simulink model "DCC_DTC_v5"  (R2023b)
settings: Solver=FixedStepDiscrete  StartTime=0.0  StopTime=0.4  MaxStep=1e-  RelTol=1e-6
undefined symbols (not defined in the file): DiscIntNeverNeededParam
libraries: spsPermanentMagnetSynchronousMachineLib x3, simulink x2, spsDCVoltageSourceLib x1, spsGroundLib x1, slpidlib x1, spsThreePhaseVIMeasurementLib x1, spsUniversalBridgeLib x1, sps_lib x1
settings Model: Creator=rainy  LastModifiedBy=rainy
settings DataIOCC: ReturnWorkspaceOutputs=off

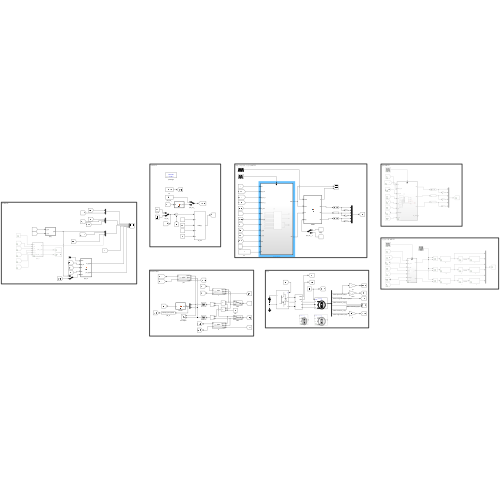
[thumbnail: Simulink's stored preview of the top-level diagram]
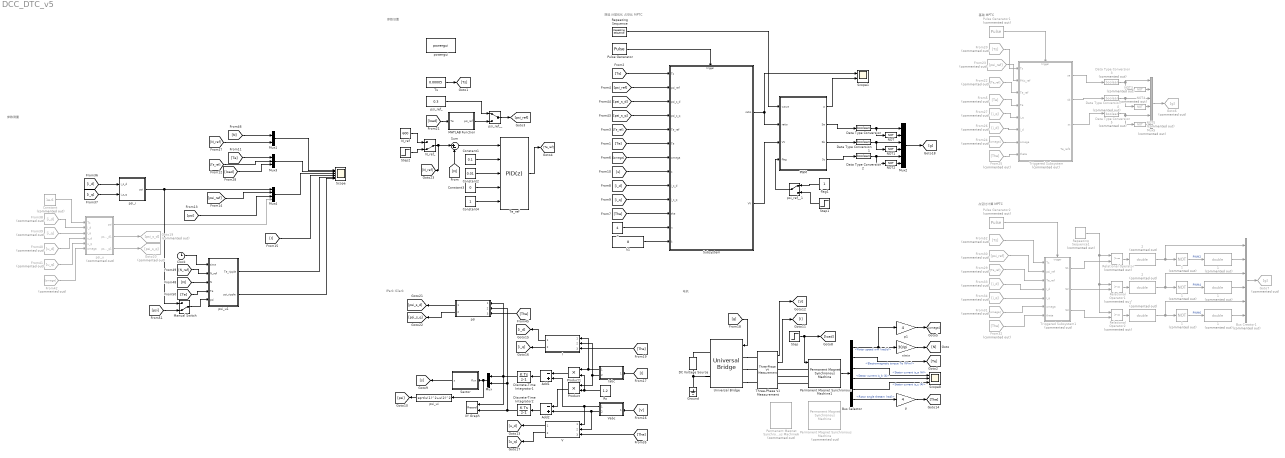
== system DCC_DTC_v5 ==
  note: 参数设置
  note: 参数测量
  note: IPark IClark
  note: 电机
  note: 基础 MPTC
  note: 占空比计算 MPTC
  note: 筛选 分层优化 占空比 MPTC
  "         1" : DataTypeConversion  Commented=on  OutDataTypeStr=double  SaturateOnIntegerOverflow=off  RndMeth=Floor
  "         2" : DataTypeConversion  Commented=on  OutDataTypeStr=double  SaturateOnIntegerOverflow=off  RndMeth=Floor
  "       1" : Logic  Commented=on  Operator=NOT  AllPortsSameDT=off  OutDataTypeStr=boolean
  "     1" : DataTypeConversion  Commented=on  OutDataTypeStr=double  SaturateOnIntegerOverflow=off  RndMeth=Floor
  "     2" : DataTypeConversion  Commented=on  OutDataTypeStr=double  SaturateOnIntegerOverflow=off  RndMeth=Floor
  "   1" : Logic  Commented=on  Operator=NOT  AllPortsSameDT=off  OutDataTypeStr=boolean
  "  1" : DataTypeConversion  Commented=on  OutDataTypeStr=double  SaturateOnIntegerOverflow=off  RndMeth=Floor
  "  2" : DataTypeConversion  Commented=on  OutDataTypeStr=double  SaturateOnIntegerOverflow=off  RndMeth=Floor
  " 1" : Logic  Commented=on  Operator=NOT  AllPortsSameDT=off  OutDataTypeStr=boolean
  Add1 : Sum  Inputs=-+
  Add2 : Sum  Inputs=-+
  Bus Creator1 : BusCreator  Commented=on  Inputs=6
  Bus Selector : BusSelector  OutputSignals=Rotor speed wm (rad/s),Electromagnetic torque Te (N*m),Stator current is_a (A),Stator current is_b (A),Stator current is_c (A),Rotor angle thetam (rad)
  Clock : Clock
  Constant : Constant  Commented=on  Value=1e-6
  Constant1 : Constant  Value=0.1
  Constant2 : Constant  Value=0.01
  Constant3 : Constant  Value=0
  Constant4 : Constant
  DC Voltage Source : spsDCVoltageSourceLib/DC Voltage Source  Amplitude=311  Measurements=Voltage
  Data Type Conversion : DataTypeConversion  OutDataTypeStr=boolean  SaturateOnIntegerOverflow=off  RndMeth=Floor
  Data Type Conversion1 : DataTypeConversion  OutDataTypeStr=boolean  SaturateOnIntegerOverflow=off  RndMeth=Floor
  Data Type Conversion2 : DataTypeConversion  OutDataTypeStr=boolean  SaturateOnIntegerOverflow=off  RndMeth=Floor
  Data Type Conversion3 : DataTypeConversion  Commented=on  OutDataTypeStr=boolean  SaturateOnIntegerOverflow=off  RndMeth=Floor
  Data Type Conversion4 : DataTypeConversion  Commented=on  OutDataTypeStr=boolean  SaturateOnIntegerOverflow=off  RndMeth=Floor
  Data Type Conversion5 : DataTypeConversion  Commented=on  OutDataTypeStr=boolean  SaturateOnIntegerOverflow=off  RndMeth=Floor
  Discrete-Time Integrator1 : DiscreteIntegrator  SampleTime=-1  ICPrevOutput=DiscIntNeverNeededParam  ICPrevScaledInput=DiscIntNeverNeededParam
  Discrete-Time Integrator2 : DiscreteIntegrator  SampleTime=-1  ICPrevOutput=DiscIntNeverNeededParam  ICPrevScaledInput=DiscIntNeverNeededParam
  From20 : From  Commented=on  GotoTag=Ts
  From22 : From  Commented=on  GotoTag=Te_ref
  From23 : From  Commented=on  GotoTag=psi_ref
  From24 : From  Commented=on  GotoTag=omega
  From25 : From  Commented=on  GotoTag=The
  From26 : From  Commented=on  GotoTag=i_d
  From27 : From  Commented=on  GotoTag=i_q
  From29 : From  Commented=on  GotoTag=Te_ref
  From30 : From  Commented=on  GotoTag=psi_ref
  From31 : From  Commented=on  GotoTag=omega
  From32 : From  Commented=on  GotoTag=The
  From33 : From  Commented=on  GotoTag=i_d
  From34 : From  Commented=on  GotoTag=i_q
  From38 : From  Commented=on  GotoTag=i_d
  From39 : From  Commented=on  GotoTag=i_q
  From40 : From  Commented=on  GotoTag=u_d
  From41 : From  Commented=on  GotoTag=u_q
  From42 : From  Commented=on  GotoTag=omega
  From5 : From  Commented=on  GotoTag=Te
  From52 : From  Commented=on  GotoTag=Ts
  Goto19 : Goto  Commented=on  GotoTag=psi_s_d
  Goto20 : Goto  Commented=on  GotoTag=psi_s_q
  Goto6 : Goto  Commented=on  GotoTag=g
  Goto7 : Goto  Commented=on  GotoTag=g
  Ground : spsGroundLib/Ground  LConnTagsString=a
  I : Subsystem  ReferencedSubsystem=Park
  Iabc : Subsystem  ReferencedSubsystem=Clark
  MATLAB Function : MATLAB Function  TreatAsAtomicUnit=on
  Manual Switch : ManualSwitch  CurrentSetting=0
  Mux : Mux  Inputs=2
  Mux1 : Mux  Inputs=2
  Mux2 : Mux  Inputs=6
  Mux3 : Mux  Inputs=3
  Mux4 : Mux
  Mux5 : Mux  Commented=on  Inputs=6
  NOT : Logic  Operator=NOT  IconShape=distinctive  AllPortsSameDT=off  OutDataTypeStr=boolean
  NOT1 : Logic  Operator=NOT  IconShape=distinctive  AllPortsSameDT=off  OutDataTypeStr=boolean
  NOT2 : Logic  Operator=NOT  IconShape=distinctive  AllPortsSameDT=off  OutDataTypeStr=boolean
  NOT3 : Logic  Commented=on  Operator=NOT  IconShape=distinctive  AllPortsSameDT=off  OutDataTypeStr=boolean
  NOT4 : Logic  Commented=on  Operator=NOT  IconShape=distinctive  AllPortsSameDT=off  OutDataTypeStr=boolean
  NOT5 : Logic  Commented=on  Operator=NOT  IconShape=distinctive  AllPortsSameDT=off  OutDataTypeStr=boolean
  N_ref : Constant  Value=600
  N_ref_ : ManualSwitch  CurrentSetting=0
  PWM : MATLAB Function  TreatAsAtomicUnit=on
  Permanent Magnet Synchronous Machine : spsPermanentMagnetSynchronousMachineLib/Permanent Magnet Synchronous Machine  Commented=on  NbPhases=3  FluxDistribution=Sinusoidal  RotorType=Salient-pole  MechanicalLoad=Torque Tm  PresetModel="02:  1.7 Nm 300 Vdc 3750 RPM - 1.7 Nm"  ShowDetailedParameters=on  MeasurementBus=off  Resistance=4.765  Inductance=8.5e-3  dqInductances=[0.0133 0.0147]  La=0.0005  MachineConstant=Flux linkage established by magnets (V.s)  Flux=0.1848  VoltageCst=67.038  TorqueCst=0.5544  Flat=120  Mechanical=[0.0001051 4.047e-05 2 0]  PolePairs=2  InitialConditions=[0 0 0 0]  InitialConditions5ph=[0 0 0 0 0 0]  RefAngle=Aligned with phase A axis (original Park)  IterativeDiscreteModel=Trapezoidal non iterative  TsBlock=-1  TsPowergui=0
  Permanent Magnet Synchronous Machine1 : spsPermanentMagnetSynchronousMachineLib/Permanent Magnet Synchronous Machine  NbPhases=3  FluxDistribution=Sinusoidal  RotorType=Round  MechanicalLoad=Torque Tm  PresetModel=No  ShowDetailedParameters=on  MeasurementBus=off  Resistance=1.2  Inductance=8.5e-3  dqInductances=[8.5e-3,8.5e-3]  La=8.5e-3  MachineConstant=Flux linkage established by magnets (V.s)  Flux=0.175  VoltageCst=126.966  TorqueCst=1.05  Flat=120  Mechanical=[0.0008 0.0004924 4 0]  PolePairs=4  InitialConditions=[0,0, 0,0]  InitialConditions5ph=[0 0 0 0 0 0]  RefAngle=Aligned with phase A axis (original Park)  IterativeDiscreteModel=Trapezoidal non iterative  TsBlock=-1  TsPowergui=0
  Permanent Magnet Synchronous Machine6 : spsPermanentMagnetSynchronousMachineLib/Permanent Magnet Synchronous Machine  Commented=on  NbPhases=3  FluxDistribution=Sinusoidal  RotorType=Round  MechanicalLoad=Torque Tm  PresetModel=No  ShowDetailedParameters=on  MeasurementBus=off  Resistance=0.25  Inductance=8.5e-3  dqInductances=[8.5e-3,8.5e-3]  La=0.0005  MachineConstant=Flux linkage established by magnets (V.s)  Flux=0.01325  VoltageCst=9.6131  TorqueCst=0.0795  Flat=120  Mechanical=[0.00003 0 4 0]  PolePairs=4  InitialConditions=[0,0, 0,0]  InitialConditions5ph=[0 0 0 0 0 0]  RefAngle=Aligned with phase A axis (original Park)  IterativeDiscreteModel=Trapezoidal non iterative  TsBlock=-1  TsPowergui=0
  Product : Product
  Product1 : Product
  Pulse Generator : DiscretePulseGenerator  PulseType=Time based  Period=0.00005
  Pulse Generator1 : DiscretePulseGenerator  Commented=on  PulseType=Time based  Period=0.00005
  Pulse Generator2 : DiscretePulseGenerator  Commented=on  PulseType=Time based  Period=0.00005
  Relational Operator : RelationalOperator  Commented=on  OutDataTypeStr=boolean  RndMeth=Simplest  InputSameDT=off
  Relational Operator1 : RelationalOperator  Commented=on  OutDataTypeStr=boolean  RndMeth=Simplest  InputSameDT=off
  Relational Operator2 : RelationalOperator  Commented=on  OutDataTypeStr=boolean  RndMeth=Simplest  InputSameDT=off
  Repeating Sequence : simulink/Sources/Repeating Sequence  rep_seq_t=[0 0.000025 0.00005]  rep_seq_y=[0 1 0]
  Repeating Sequence1 : simulink/Sources/Repeating Sequence  Commented=on  rep_seq_t=[0 0.000025 0.00005]  rep_seq_y=[0 0.000025 0]
  Rs : Constant  Value=1.2
  Scope : Scope  NumInputPorts=6
  Scope1 : Scope  NumInputPorts=2
  Scope8 : Scope  NumInputPorts=3
  Sector : MATLAB Function  TreatAsAtomicUnit=on
  Step : Step  Time=0.2  After=0  SampleTime=0
  Step1 : Step  Time=0.1  SampleTime=0
  Step2 : Step  Time=0.2  Before=400  After=600  SampleTime=0
  Subsystem : Subsystem
  Sum : Sum  Inputs=|+-
  Te_ref : slpidlib/PID Controller  Controller=PID  Form=Parallel  TimeDomain=Discrete-time  UseExternalTs=off  SampleTime=-1  IntegratorMethod=Forward Euler  FilterMethod=Forward Euler  ControllerParametersSource=external  P=1  I=1  UseKiTs=off  D=0  N=100  UseFilter=on  TunerSelectOption=Transfer Function Based (PID Tuner App)  InitialConditionSource=internal  InitialConditionForIntegrator=0  InitialConditionForFilter=0  DifferentiatorICPrevScaledInput=0  ExternalReset=none  TrackingMode=off  Kt=1  LimitOutput=off  SatLimitsSource=internal  UpperSaturationLimit=inf  LowerSaturationLimit=-inf  LinearizeAsGain=off  AntiWindupMode=none  Kb=1  LimitIntegrator=off  UpperIntegratorSaturationLimit=inf  LowerIntegratorSaturationLimit=-inf  POutMin=[]  POutMax=[]  IOutMin=[]  IOutMax=[]  DOutMin=[]  DOutMax=[]  NOutMin=[]  NOutMax=[]  SumOutMin=[]  SumOutMax=[]  SaturationOutMin=[]  SaturationOutMax=[]  PParamMin=[]  PParamMax=[]  IParamMin=[]  IParamMax=[]  DParamMin=[]  DParamMax=[]  NParamMin=[]  NParamMax=[]  KbParamMin=[]  KbParamMax=[]  KtParamMin=[]  KtParamMax=[]  KbOutMin=[]  KbOutMax=[]  KtOutMin=[]  KtOutMax=[]  IntegratorOutMin=[]  IntegratorOutMax=[]  FilterOutMin=[]  FilterOutMax=[]  SumI1OutMin=[]  SumI1OutMax=[]  SumI2OutMin=[]  SumI2OutMax=[]  SumI3OutMin=[]  SumI3OutMax=[]  SumI4OutMin=[]  SumI4OutMax=[]  SumDOutMin=[]  SumDOutMax=[]  DifferentiatorOutMin=[]  DifferentiatorOutMax=[]  FilterDiffOutCoefMin=[]  FilterDiffOutCoefMax=[]  ReciprocalOutMin=[]  ReciprocalOutMax=[]  SumDenOutMin=[]  SumDenOutMax=[]  SumNumOutMin=[]  SumNumOutMax=[]  DivideOutMin=[]  DivideOutMax=[]  UdiffTsProdOutMin=[]  UdiffTsProdOutMax=[]  NTsProdOutMin=[]  NTsProdOutMax=[]  UintegralTsProdOutMin=[]  UintegralTsProdOutMax=[]  UngainTsProdOutMin=[]  UngainTsProdOutMax=[]  ClampingZeroOutDataTypeStr=Inherit: Inherit via back propagation  ClampingZeroOutMin=[]  ClampingZeroOutMax=[]  FilterDenConstantOutDataTypeStr=Inherit: Inherit via back propagation  FilterDenConstantOutMin=[]  FilterDenConstantOutMax=[]  PCopyOutDataTypeStr=Inherit: Inherit via back propagation  PCopyOutMin=[]  PCopyOutMax=[]  NCopyOutDataTypeStr=Inherit: Inherit via back propagation  NCopyOutMin=[]  NCopyOutMax=[]  IntegratorContinuousStateAttributes=''  IntegratorStateMustResolveToSignalObject=off  IntegratorRTWStateStorageClass=Auto  FilterContinuousStateAttributes=''  FilterStateMustResolveToSignalObject=off  FilterRTWStateStorageClass=Auto  ParallelPVariant=ExternalParameters  IdealPVariant=Disabled  IVariant=ExternalParameters  DVariant=ExternalParameters  IntegratorVariant=Discrete  SatVariant=Disabled  AWVariant=Passthrough  PCopyVariant=Disabled  TRVariant=Disabled  FdbkBlocksVariant=Forward  IdealPFdbkVariant=Disabled  SatFdbkVariant=Disabled  DerivativeFilterVariant=ForwardEulerFilter  NVariant=ExternalParameters  NCopyVariant=Disabled  FilterICVariant=InternalICsFilter  IntegratorICVariant=InternalICs  ExternalResetVariant=Disabled  TRSumVariant=Passthrough  SumFdbkVariant=Disabled  SumVariant=Sum_PID  TsampFilterVariant=InternalTs  TsampNgainVariant=Passthrough  TsampIntegralVariant=Disabled_SignalSpec  ExternalSaturationOutDataTypeStr=Inherit: Same as second input
      settings: LibrarySourceBlock=simulink/Discrete/Discrete PID Controller
  Three-Phase V-I Measurement : spsThreePhaseVIMeasurementLib/Three-Phase V-I Measurement  VoltageMeasurement=phase-to-ground  SetLabelV=off  LabelV=Vabc  Vpu=off  VpuLL=off  CurrentMeasurement=yes  SetLabelI=off  LabelI=Iabc  Ipu=off  Pbase=100e6  Vbase=500e3  OutputType=Complex  PhasorSimulation=off  PSBequivalent=0
  Triggered Subsystem : Subsystem  Commented=on  TreatAsAtomicUnit=on
  Triggered Subsystem1 : Subsystem  Commented=on  TreatAsAtomicUnit=on
  Ts : Constant  Value=0.00005
  Universal Bridge : spsUniversalBridgeLib/Universal Bridge  Arms=3  SnubberResistance=1e5  SnubberCapacitance=inf  Device=IGBT / Diodes  Ron=1e-3  Lon=0  ForwardVoltages="[  0  0  ]"  ForwardVoltage=0  GTOparameters=[ 10e-6 , 20e-6 ]  IGBTparameters=[ 1e-6 , 2e-6 ]  Measurements=None  Measurements_2=None  converterType=Rectifier
  V : Subsystem  ReferencedSubsystem=Park
  Vabc : Subsystem  ReferencedSubsystem=Clark
  XY Graph : Record  FileSettingsInternal="{\"entries\":[{\"content\":{\"excelSettings\":{\"content\":{},\"type\":\"Streamout.ExcelSettings\"}},\"type\":\"Streamout.FileSettingStorage\",\"uuid\":\"\"}],\"packageUris\":[\"http:\\/\\/schema.mathworks.com\\/mf0\\/streamout_blocks\\/R2020a\"],\"version\":\"1.0\"}"  Layout=[1 1]  SignalsInternal="{\"entries\":[{\"content\":{\"signals\":[{\"content\":{\"blockPath\":[],\"dimensions\":[1],\"domain\":\"\",\"lineColor\":\"#a2142f\",\"plots\":[1],\"port\":1,\"sid\":[\"\"],\"signalID\":316,\"signalName\":\"Discrete-Time\\nIntegrator1\"},\"type\":\"RecordBlkView.Signal\",\"uuid\":\"\"},{\"content\":{\"blockPath\":[],\"dimensions\":[1],\"domain\":\"\",\"lineColor\":\"#139fff\",\"plots\":[1],\"port\":2,\"sid\":[\"\"],\"signalID\":320,\"signalName\":\"Discrete-Time\\nIntegrator2\"},\"type\":\"RecordBlkView.Signal\",\"uuid\":\"\"}]},\"type\":\"RecordBlkView.InputSignals\",\"uuid\":\"\"}],\"packageUris\":[\"http:\\/\\/schema.mathworks.com\\/mf0\\/streamout_blocks\\/R2020a\"],\"version\":\"1.0\"}"  VisualizationBindings="{\"xyplotplugin\":{\"info\":[{\"series\":[{\"bindingParametersList\":[{\"parameter\":\"X-Axis\",\"signalID\":316,\"signalName\":\"Discrete-Time\\nIntegrator1\"},{\"parameter\":\"Y-Axis\",\"signalID\":320,\"signalName\":\"Discrete-Time\\nIntegrator2\"}],\"seriesID\":39498}],\"subplotID\":1}]}}"  CompatibilityTag=XY  st=-1
  flag1 : Constant
  k1 : Constant  Value=8
  n : Constant  Value=4
  p : Gain  Gain=4
  p1 : Gain  Gain=4
  powergui : sps_lib/powergui  Priority=1  SimulationMode=Discrete  SampleTime=1e-6  frequency=60  Iterations=50  frequencyindice=0  Pbase=100e6  ErrMax=1e-4  UnitsV=kV  UnitsW=MW  buscounter=0  FunctionMessages=off  echomessages=off  EnableUseOfTLC=off  CurrentSourceSwitches=off  DisableSnubberDevices=off  DisableRonSwitches=off  DisableVfSwitches=off  DisplayEquations=off  AutomaticDiscreteSolvers=off  SolverType=Tustin/Backward Euler (TBE)  Interpol=off  ExternalGateDelay=off  methode=off  Ts=100  x0status=blocks  SPID=on  SwTol=0  HookPort=off  NonlinearTolerance=1e-4  nMaxIteration=100  ContinueOnMaxIteration=off  RestoreLinks=warning  ResistiveCurrentMeasurement=off  Frange=[0:2:500]  Ylog=off  Xlog=on  ShowGrid=off  save=off  variable=ZData  structure=0  ZoomFFT=off  StartTime=0.0  cycles=1  DisplayStyle=1  fundamental=60  FreqAxis=off  MaxFrequency=1000  frequencyindicesteady=1  RmsSteady=1  display=off
  psi : Subsystem  ReferencedSubsystem=Park
  psi_i : MATLAB Function  TreatAsAtomicUnit=on
  psi_ref_ : Constant  Value=0.3
  psi_ref__ : ManualSwitch
  psi_ref__1 : ManualSwitch
  psi_u : MATLAB Function  Commented=on  TreatAsAtomicUnit=on
  psi_u1 : MATLAB Function  TreatAsAtomicUnit=on
  psi_ui : Fcn  Expr=sqrt(u(1)^2+u(2)^2)
  r/min : Gain  Gain=30/pi
  wires:
  N_ref_/1 -> [N_ref], Sum/1
  Sum/1 -> Te_ref/1
  Bus Selector/1 -> p1/1, r/min/1  "<Rotor speed wm (rad/s)>"
  r/min/1 -> [N]
  [N] -> Sum/2
  NOT1/1 -> Mux2/4
  Data Type Conversion2/1 -> NOT2/1, Mux2/5
  NOT2/1 -> Mux2/6
  Data Type Conversion/1 -> NOT/1, Mux2/1
  NOT/1 -> Mux2/2
  Data Type Conversion1/1 -> NOT1/1, Mux2/3
  Iabc/1 -> I/1, Product1/1
  Iabc/2 -> Product/1, I/2
  Rs/1 -> Product/2, Product1/2
  Product1/1 -> Add1/1
  Vabc/1 -> V/1, Add1/2
  Product/1 -> Add2/1
  Vabc/2 -> V/2, Add2/2
  Add2/1 -> Discrete-Time Integrator2/1
  Add1/1 -> Discrete-Time Integrator1/1
  Ts/1 -> [Ts]
  Mux/1 -> psi_ui/1, Sector/1(flux)
  Bus Selector/2 -> [Te]  "<Electromagnetic torque Te (N*m)>"
  [Te] -> Subsystem/6(Te)
  Three-Phase V-I Measurement/2 -> [I]
  PWM/4(Sc) -> Data Type Conversion2/1
  PWM/3(Sb) -> Data Type Conversion1/1
  PWM/2(Sa) -> Data Type Conversion/1
  [Ts] -> Subsystem/1(Ts)
  [psi_ref] -> Subsystem/2(psi_ref)
  Repeating Sequence/1 -> PWM/1(wave)
  Pulse Generator/1 -> Subsystem/Trigger
  n/1 -> Subsystem/12(n)
  Bus Selector/3 -> Scope8/1  "<Stator current is_a (A)>"
  Bus Selector/4 -> Scope8/2  "<Stator current is_b (A)>"
  Bus Selector/5 -> Scope8/3  "<Stator current is_c (A)>"
  Step/1 -> Permanent Magnet Synchronous Machine1/1, [load]
  Subsystem/1(ratio) -> Scope1/1, PWM/2(ratio)
  Subsystem/2(VV) -> PWM/3(VV)
  Te_ref/1 -> [Te_ref]
  [Te_ref] -> Subsystem/5(Te_ref)
  [omega] -> Subsystem/7(omega)
  [i_d] -> Subsystem/9(i_s_d)
  [i_q] -> Subsystem/10(i_s_q)
  Sector/1(s) -> [s]
  [s] -> Subsystem/8(s)
  PWM/1(w) -> Scope1/2
  psi_ui/1 -> [psi]
  Mux1/1 -> Scope/1
  Mux3/1 -> Scope/2
  Mux4/1 -> Scope/3
  [I] -> Scope/4
  [Te] -> Mux3/1
  [psi_ref] -> Mux4/2
  Three-Phase V-I Measurement/1 -> [V]
  [I] -> Iabc/1
  [V] -> Vabc/1
  Mux2/1 -> [g]
  [g] -> Universal Bridge/1
  Bus Selector/6 -> p/1  "<Rotor angle thetam (rad)>"
  p/1 -> [The]
  [The] -> I/3
  I/2 -> [i_q]
  I/1 -> [i_d]
  p1/1 -> [omega]
  k1/1 -> Subsystem/13(k)
  Discrete-Time Integrator1/1 -> psi/1, XY Graph/1, Mux/1
  Discrete-Time Integrator2/1 -> XY Graph/2, psi/2, Mux/2
  [load] -> MATLAB Function/1(Te)
  psi_ref_/1 -> psi_ref__/1
  MATLAB Function/1(psi_ref) -> psi_ref__/2
  psi_ref__/1 -> [psi_ref]
  [i_d] -> psi_i/1(i_s_d)
  [i_q] -> psi_i/2(i_s_q)
  Permanent Magnet Synchronous Machine1/1 -> Bus Selector/1
  [psi] -> Mux4/3
  [The] -> Subsystem/11(the)
  NOT3/1 -> Mux5/2
  NOT4/1 -> Mux5/4
  NOT5/1 -> Mux5/6
  Triggered Subsystem/1(sa) -> Data Type Conversion3/1
  Data Type Conversion5/1 -> NOT5/1, Mux5/5
  Triggered Subsystem/2(sb) -> Data Type Conversion4/1
  Triggered Subsystem/3(sc) -> Data Type Conversion5/1
  Data Type Conversion3/1 -> NOT3/1, Mux5/1
  Data Type Conversion4/1 -> NOT4/1, Mux5/3
  Mux5/1 -> Goto6/1
  From25/1 -> Triggered Subsystem/8(theta)
  From24/1 -> Triggered Subsystem/7(omega)
  From26/1 -> Triggered Subsystem/6(i_d)
  From27/1 -> Triggered Subsystem/5(i_q)
  From5/1 -> Triggered Subsystem/4(Te)
  From22/1 -> Triggered Subsystem/3(Te_ref)
  From23/1 -> Triggered Subsystem/2(Phis_ref)
  From20/1 -> Triggered Subsystem/1(Ts)
  Pulse Generator1/1 -> Triggered Subsystem/Trigger
  [load] -> Mux3/3
  [Te_ref] -> Mux3/2
  flag1/1 -> psi_ref__1/1
  Step1/1 -> psi_ref__1/2
  psi_ref__1/1 -> PWM/4(flag)
  From30/1 -> Triggered Subsystem1/2(psi_ref)
  From29/1 -> Triggered Subsystem1/3(Te_ref)
  From34/1 -> Triggered Subsystem1/5(i_q)
  From33/1 -> Triggered Subsystem1/4(i_d)
  From31/1 -> Triggered Subsystem1/6(omega)
  From32/1 -> Triggered Subsystem1/7("theta ")
  [The] -> V/3
  V/1 -> [u_d]
  V/2 -> [u_q]
  Constant/1 -> psi_u/1(Ts)
  From40/1 -> psi_u/4(u_d)
  From41/1 -> psi_u/5(u_q)
  psi_u/1(psi) -> Mux4/4
  From42/1 -> psi_u/6(omega)
  psi_u/2(psi_s_d1) -> Goto19/1
  psi_u/3(psi_s_q1) -> Goto20/1
  [psi_s_d] -> Subsystem/3(psi_s_d)
  [psi_s_q] -> Subsystem/4(psi_s_q)
  psi/1 -> [psi_s_d]
  psi/2 -> [psi_s_q]
  [The] -> psi/3
  Constant1/1 -> Te_ref/2
  Constant2/1 -> Te_ref/3
  Constant3/1 -> Te_ref/4
  Constant4/1 -> Te_ref/5
  N_ref/1 -> N_ref_/1
  Step2/1 -> N_ref_/2
  [N_ref] -> Mux1/2
  [N] -> Mux1/1
  From39/1 -> psi_u/3(i_q)
  From38/1 -> psi_u/2(i_d)
  [N_ref] -> psi_u1/2(N_ref)
  [N] -> psi_u1/3(N)
  [Te] -> psi_u1/4(Te)
  psi_u1/1(Te_ripple) -> Scope/5
  psi_u1/2(psi_ripple) -> Scope/6
  From52/1 -> Triggered Subsystem1/1(Ts)
  Pulse Generator2/1 -> Triggered Subsystem1/Trigger
  Triggered Subsystem1/1(S1) -> Relational Operator/2
  Triggered Subsystem1/2(S2) -> Relational Operator1/2
  "  2"/1 -> Bus Creator1/1, " 1"/1
  Bus Creator1/1 -> Goto7/1
  Relational Operator/1 -> "  2"/1
  "         1"/1 -> Bus Creator1/6
  Relational Operator2/1 -> "         2"/1
  "       1"/1 -> "         1"/1  "PWM6"
  Relational Operator1/1 -> "     2"/1
  "   1"/1 -> "     1"/1  "PWM4"
  " 1"/1 -> "  1"/1  "PWM2"
  "  1"/1 -> Bus Creator1/2
  Repeating Sequence1/1 -> Relational Operator2/1, Relational Operator1/1, Relational Operator/1
  "         2"/1 -> Bus Creator1/5, "       1"/1
  "     1"/1 -> Bus Creator1/4
  "     2"/1 -> Bus Creator1/3, "   1"/1
  Triggered Subsystem1/3(S3) -> Relational Operator2/2
  Clock/1 -> psi_u1/1(time)
  Manual Switch/1 -> psi_u1/5(psi)
  [psi] -> Manual Switch/2
  psi_i/1(psi) -> Manual Switch/1, Mux4/1
  connections:
  Universal Bridge/RConn2 -- DC Voltage Source/LConn1 -- Ground/LConn1
  Universal Bridge/LConn3 -- Three-Phase V-I Measurement/LConn3
  Universal Bridge/LConn1 -- Three-Phase V-I Measurement/LConn1
  Universal Bridge/LConn2 -- Three-Phase V-I Measurement/LConn2
  DC Voltage Source/RConn1 -- Universal Bridge/RConn1
  Permanent Magnet Synchronous Machine1/LConn1 -- Three-Phase V-I Measurement/RConn1
  Permanent Magnet Synchronous Machine1/LConn2 -- Three-Phase V-I Measurement/RConn2
  Permanent Magnet Synchronous Machine1/LConn3 -- Three-Phase V-I Measurement/RConn3

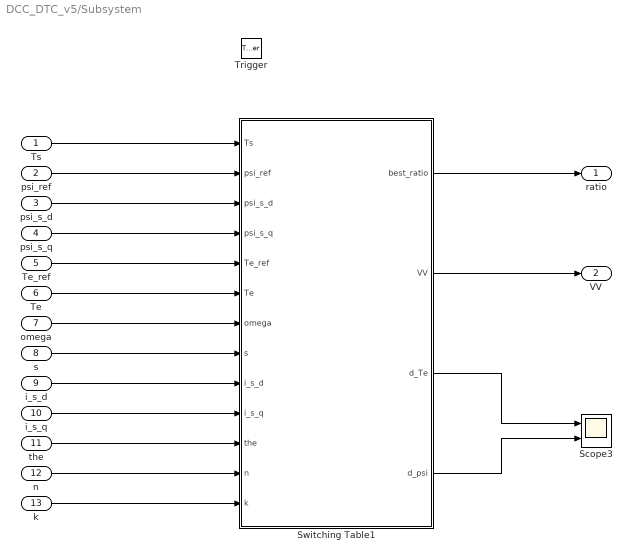
== system DCC_DTC_v5/Subsystem ==
  Ts : Inport
  psi_ref : Inport  Port=2
  psi_s_d : Inport  Port=3
  psi_s_q : Inport  Port=4
  Te_ref : Inport  Port=5
  Te : Inport  Port=6
  omega : Inport  Port=7
  s : Inport  Port=8
  i_s_d : Inport  Port=9
  i_s_q : Inport  Port=10
  the : Inport  Port=11
  n : Inport  Port=12
  k : Inport  Port=13
  Trigger : TriggerPort  VariantControl=(inherit)  PortDimensions=1
  Scope3 : Scope  NumInputPorts=2
  Switching Table1 : MATLAB Function  TreatAsAtomicUnit=on
  ratio : Outport
  VV : Outport  Port=2
  wires:
  Ts/1 -> Switching Table1/1(Ts)
  psi_ref/1 -> Switching Table1/2(psi_ref)
  Te_ref/1 -> Switching Table1/5(Te_ref)
  Te/1 -> Switching Table1/6(Te)
  omega/1 -> Switching Table1/7(omega)
  s/1 -> Switching Table1/8(s)
  i_s_q/1 -> Switching Table1/10(i_s_q)
  Switching Table1/1(best_ratio) -> ratio/1
  k/1 -> Switching Table1/13(k)
  n/1 -> Switching Table1/12(n)
  Switching Table1/2(VV) -> VV/1
  i_s_d/1 -> Switching Table1/9(i_s_d)
  Switching Table1/4(d_psi) -> Scope3/2
  the/1 -> Switching Table1/11(the)
  Switching Table1/3(d_Te) -> Scope3/1
  psi_s_d/1 -> Switching Table1/3(psi_s_d)
  psi_s_q/1 -> Switching Table1/4(psi_s_q)

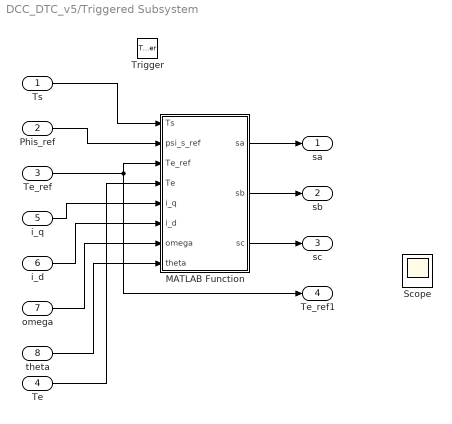
== system DCC_DTC_v5/Triggered Subsystem ==
  Ts : Inport
  Phis_ref : Inport  Port=2
  Te_ref : Inport  Port=3
  Te : Inport  Port=4
  i_q : Inport  Port=5
  i_d : Inport  Port=6
  omega : Inport  Port=7
  theta : Inport  Port=8
  Trigger : TriggerPort  VariantControl=(inherit)
  MATLAB Function : MATLAB Function  TreatAsAtomicUnit=on
  Scope : Scope  NumInputPorts=2
  sa : Outport
  sb : Outport  Port=2
  sc : Outport  Port=3
  Te_ref1 : Outport  Port=4
  wires:
  Phis_ref/1 -> MATLAB Function/2(psi_s_ref)
  Te_ref/1 -> Te_ref1/1, MATLAB Function/3(Te_ref)
  i_q/1 -> MATLAB Function/5(i_q)
  i_d/1 -> MATLAB Function/6(i_d)
  omega/1 -> MATLAB Function/7(omega)
  theta/1 -> MATLAB Function/8(theta)
  MATLAB Function/1(sa) -> sa/1
  MATLAB Function/2(sb) -> sb/1
  MATLAB Function/3(sc) -> sc/1
  Ts/1 -> MATLAB Function/1(Ts)
  Te/1 -> MATLAB Function/4(Te)
  ? -> Scope/1
  ? -> Scope/2

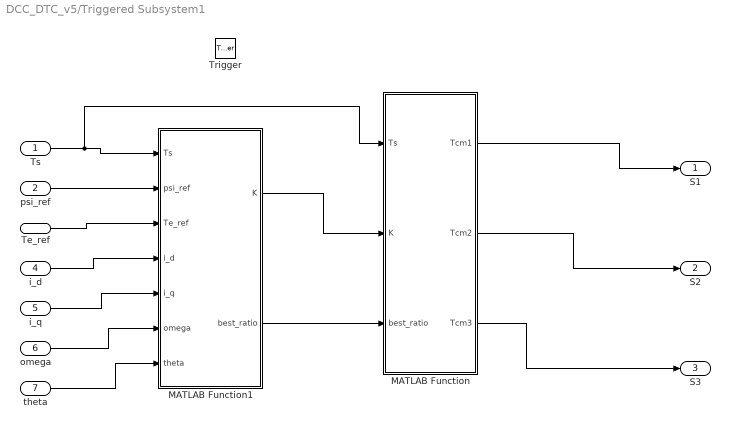
== system DCC_DTC_v5/Triggered Subsystem1 ==
  Ts : Inport
  psi_ref : Inport  Port=2
  Te_ref : Inport  Port=3
  i_d : Inport  Port=4
  i_q : Inport  Port=5
  omega : Inport  Port=6
  "theta " : Inport  Port=7
  Trigger : TriggerPort  VariantControl=(inherit)
  MATLAB Function : MATLAB Function  TreatAsAtomicUnit=on
  MATLAB Function1 : MATLAB Function  TreatAsAtomicUnit=on
  S1 : Outport  VectorParamsAs1DForOutWhenUnconnected=off
  S2 : Outport  Port=2  VectorParamsAs1DForOutWhenUnconnected=off
  S3 : Outport  Port=3  VectorParamsAs1DForOutWhenUnconnected=off
  wires:
  Ts/1 -> MATLAB Function/1(Ts), MATLAB Function1/1(Ts)
  psi_ref/1 -> MATLAB Function1/2(psi_ref)
  "theta "/1 -> MATLAB Function1/7(theta)
  omega/1 -> MATLAB Function1/6(omega)
  i_q/1 -> MATLAB Function1/5(i_q)
  i_d/1 -> MATLAB Function1/4(i_d)
  Te_ref/1 -> MATLAB Function1/3(Te_ref)
  MATLAB Function1/2(best_ratio) -> MATLAB Function/3(best_ratio)
  MATLAB Function/1(Tcm1) -> S1/1
  MATLAB Function/2(Tcm2) -> S2/1
  MATLAB Function/3(Tcm3) -> S3/1
  MATLAB Function1/1(K) -> MATLAB Function/2(K)

== matlab function DCC_DTC_v5/psi_u ==
  data: psi output; Ts input; i_d input; i_q input; psi_s_d1 output; u_d input; u_q input; psi_s_q1 output; omega input
function [psi, psi_s_d1, psi_s_q1]  = fcn(Ts, i_d, i_q, u_d, u_q, omega)

p = 4;
R_s = 1.2;
L_d = 0.0085;
L_q = 0.0085;
V = 311;
psi_f = 0.175;

ratio = 1;

persistent M psi_s_d psi_s_q 
if isempty(M)
    M=1; 
    psi_s_d = 0;  
    psi_s_q = 0; 
end

psi_s_d1 = (1-Ts*R_s/L_d)*psi_s_d + (0+Ts*omega)*psi_s_q + ratio*Ts*u_d + R_s*Ts/L_d*psi_f;
psi_s_q1 = (0-Ts*omega)*psi_s_d + (1-Ts*R_s/L_q)*psi_s_q + ratio*Ts*u_q + R_s*Ts/L_d*0;

psi = sqrt(psi_s_d^2+psi_s_q^2);

psi_s_d = psi_s_d1;
psi_s_q = psi_s_q1;

== matlab function DCC_DTC_v5/psi_i ==
  data: i_s_d input; i_s_q input; psi output
function psi = fcn(i_s_d, i_s_q)

% 给定的参数值
p = 4;
R_s = 1.2;
L_d = 0.0085;
L_q = 0.0085;
V = 311;
psi_f = 0.175;

psi_r = psi_f + 1i*0;
psi_s_d = L_d*i_s_d + psi_f;
psi_s_q = L_q*i_s_q;

i_s = i_s_d + 1i*i_s_q;
psi_s = psi_s_d + 1i*psi_s_q;


% 计算零电压矢量下变化率
psi = sqrt(psi_s_d^2 +psi_s_q^2);

== matlab function DCC_DTC_v5/psi_u1 ==
  data: time input; Te_ripple output; N_ref input; N input; Te input; psi_ripple output; psi input
function [Te_ripple, psi_ripple]  = fcn(time, N_ref, N, Te, psi)

k = 0.05;

Te_ripple = 0;
psi_ripple = 0;

persistent F M Te_max Te_min psi_max psi_min
if isempty(F)
    F = 0;
    M = 0;
    Te_max = -Inf;
    Te_min = Inf;
    psi_max = -Inf;
    psi_min = Inf;
end

% if N>N_ref*(1-k*0.1) && N<N_ref*(1+k*0.1)
%     M = 1;
% else
%     if N<N_ref*(1-k) || N>N_ref*(1+k)
%         M = 0;
%         Te_max = -Inf;
%         Te_min = Inf;
%         psi_max = -Inf;
%         psi_min = Inf;
%     end
% end

if (time>0.05 && time<0.2) || (time>0.25 && time<0.4)
    M = 1;
else
    if N<N_ref*(1-k) || N>N_ref*(1+k)
        M = 0;
        Te_max = -Inf;
        Te_min = Inf;
        psi_max = -Inf;
        psi_min = Inf;
    end
end   

if M == 1
    if Te>Te_max
        Te_max = Te;
    end
    if Te<Te_min
        Te_min = Te;
    end
    if psi>psi_max
        psi_max = psi;
    end
    if psi<psi_min
        psi_min = psi;
    end
    Te_ripple = Te_max - Te_min;
    psi_ripple = psi_max - psi_min;
end

== matlab function DCC_DTC_v5/Sector ==
  data: flux input; s output
function s = fcn(flux)

% 将\psi_{\aplha}和\psi_{\beta}分解为三相
a1 = flux(1);
b1 = flux(1)*(-0.5) + sqrt(3)/2*flux(2);
c1 = flux(1)*(-0.5) - sqrt(3)/2*flux(2);

% a1 > 0，有扇区126
% b1 > 0，有扇区234
% c1 > 0，有扇区456
% n为a1 b1 c1中>0的个数，0 < n < 3
% 
% a b c | s
%-------|---
% 1 1 0 | 2
% 1 0 1 | 6
% 1 0 0 | 1
% 0 1 1 | 4
% 0 1 0 | 3
% 0 0 1 | 5

if(flux(2) == 0)
    N = 4;
else
    if(a1 > 0)
        a = 1;
    else
        a = 0;
    end
    
    if(b1 > 0)
        b = 1;
    else
        b = 0;
    end
    
    if(c1 > 0)
        c = 1;
    else
        c = 0;
    end
    
    N = 4*a+2*b+c;
end

% if(N==0 || N==7)
%     N = 4;
% end

Sector_table=[5 3 4 1 6 2];

s = Sector_table(N);

== matlab function DCC_DTC_v5/Triggered Subsystem1/MATLAB Function1 ==
  data: Ts input; K output; psi_ref input; Te_ref input; i_d input; i_q input; omega input; theta input; best_ratio output
function [K, best_ratio] = fcn(Ts, psi_ref, Te_ref, i_d, i_q, omega, theta)

p = 4;
R_s = 1.2;
L_d = 0.0085;
L_q = 0.0085;
V = 311;
psi_f = 0.175;
g_min=Inf;
m=250;
K=1;
best_ratio=1;

sw=[0 0 0;1 0 0;1 1 0;0 1 0;0 1 1;0 0 1;1 0 1;1 1 1];
trans=2/3*[cos(theta) cos(theta-2*pi/3) cos(theta+2*pi/3);-sin(theta) -sin(theta-2*pi/3) -sin(theta+2*pi/3)];


persistent M u_d u_q 
if isempty(M)
    M=1; 
    u_d=0;  
    u_q=0; 
end

% i_q1=i_q+Ts/L_d*(u_q-i_d*omega*L_d-i_q*R_s-psi_f*omega);
% i_d1=i_d+Ts/L_q*(u_d+i_q*omega*L_q-i_d*R_s);
i_q1=i_q;
i_d1=i_d;
Te=3/2*p*i_q1*psi_f;
for i=1:8
      sa=sw(i,1);sb=sw(i,2);sc=sw(i,3);
      Va=(V*(2*sa-sb-sc))/3;
      Vb=(V*(2*sb-sa-sc))/3;   
      Vc=(V*(2*sc-sb-sa))/3;
      Vabc=[Va;Vb;Vc];
      V_dq=trans*Vabc;
      V_d=V_dq(1,1);
      V_q=V_dq(2,1);
      i_d_=1/L_d*(V_d-R_s*i_d1+omega*L_q*i_q1)*Ts;
      i_q_=1/L_q*(V_q-R_s*i_q1-omega*(psi_f+L_d*i_d1))*Ts;
      i_d2=i_d1+i_d_;
      i_q2=i_q1+i_q_;
      Te2=3/2*p*i_q2*psi_f;
      psi_s_d2=L_d*i_d2+psi_f;
      psi_s_q2=L_q*i_q2;
      psi2=sqrt(psi_s_d2^2+psi_s_q2^2);
      
      k_Te_0=1/L_q*(-R_s*i_q1-omega*(psi_f+L_d*i_d1))*(3/2*p*psi_f);
      k_Te_1=1/L_q*(V_q-R_s*i_q1-omega*(psi_f+L_d*i_d1))*(3/2*p*psi_f);
      ratio=(Te_ref-Te-k_Te_0*Ts)/(k_Te_1-k_Te_0)/Ts;
      
      if(ratio<=0||ratio>=1)
          D_flag=100000;
          ratio=1;
      else
          D_flag=0;
      end
      
      g=abs(Te_ref-Te2)+m*abs(psi_ref-psi2)+D_flag;
     
       if(g<g_min)
        K=i;
        best_ratio=ratio;
        g_min=g;
      end
end

sa=sw(K,1);sb=sw(K,2);sc=sw(K,3);
Va_min=(V*(2*sa-sb-sc))/3;
Vb_min=(V*(2*sb-sa-sc))/3;   
Vc_min=(V*(2*sc-sb-sa))/3;
Vabc_min=[Va_min;Vb_min;Vc_min];
V_dq_min=trans*Vabc_min;
u_d=V_dq_min(1,1)*best_ratio;
u_q=V_dq_min(2,1)*best_ratio;

== matlab function DCC_DTC_v5/PWM ==
  data: w output; wave input; ratio input; VV input; Sa output; Sb output; Sc output; flag input
function [w, Sa, Sb, Sc] = fcn(wave, ratio, VV, flag)

sw = [1 0 0; 1 1 0; 0 1 0; 0 1 1; 0 0 1; 1 0 1];

if(VV<1 || VV>6)
    VV = 1;
end

if(wave >= 1 - ratio || flag == 0)
    Sa= sw(VV, 1);
    Sb= sw(VV, 2);
    Sc= sw(VV, 3);
    w = 1;
else
    Sa = 0;
    Sb = 0;
    Sc = 0;
    w = 0;
end

== matlab function DCC_DTC_v5/Subsystem/Switching Table1 ==
  data: best_ratio output; Ts input; psi_ref input; psi_s_d input; psi_s_q input; Te_ref input; Te input; VV output; omega input; s input; i_s_d input; i_s_q input; the input; n input; k input; d_Te output; d_psi output
function [best_ratio, VV, d_Te, d_psi]= fcn(Ts, psi_ref, psi_s_d, psi_s_q, Te_ref, Te, omega, s, i_s_d, i_s_q, the, n, k)

% 给定的参数值
p = 4;
R_s = 1.2;
L_d = 0.0085;
L_q = 0.0085;
V = 311;
psi_f = 0.175;

psi_r = psi_f + 1i*0;
i_s = i_s_d + 1i*i_s_q;
psi_s = psi_s_d + 1i*psi_s_q;


% 计算零电压矢量下变化率
psi = sqrt(psi_s_d^2 +psi_s_q^2);
k_psi_0 = -R_s/psi*real(psi_s'*i_s); % 零电压矢量时磁链变化率
% k_psi_1 = 1/psi*real(psi_s'*u_s) + k_psi_0; % 非零电压矢量时磁链变化率

k_Te_0 = -3/2*p*(1/L_q-1/L_d)*omega*real(psi_s^2) + ...
    3/4*p*R_s*(1/L_d^2-1/L_q^2)*imag(psi_s^2) - ...
    3/2*p/L_d*(R_s/L_d*imag(psi_s*psi_r) + omega*real(psi_s*psi_r)); % 零电压矢量时转矩变化率
% k_Te_1 = 3/2*p*(1/L_q-1/L_d)*imag(u_s*psi_s) + 3/2*p/L_d*imag(u_s*psi_r) + k_Te_0;  % 非零电压矢量时转矩变化率



% 选择电压矢量
Te1 = Te + k_Te_0*Ts;
psi1 = psi + k_psi_0*Ts;

if(Te_ref > Te1)
    if(psi_ref > psi)
        VV = s+1;
    else
        VV = s+2;
    end
else
    if(psi_ref > psi)
        VV = s-1;
    else
        VV = s-2;
    end
end

if(VV < 1)
    VV = VV+6;
end
if(VV > 6)
    VV = VV-6;
end


% MPTC
sw = [1 0 0; 1 1 0; 0 1 0; 0 1 1; 0 0 1; 1 0 1];
sa = sw(VV,1); sb = sw(VV, 2); sc = sw(VV, 3);
Va = V*(2*sa-sb-sc)/3;
Vb = V*(2*sb-sc-sa)/3;
Vc = V*(2*sc-sa-sb)/3;
Vabc = [Va; Vb; Vc];
trans = 2/3*[cos(the) cos(the-2/3*pi) cos(the+2/3*pi);
             -sin(the) -sin(the-2/3*pi) -sin(the+2/3*pi)];
V_dq = trans*Vabc;
u_s = V_dq(1) + 1i*V_dq(2);

k_psi_1 = 1/psi*real(psi_s'*u_s) + k_psi_0; % 非零电压矢量时磁链变化率
k_Te_1 = 3/2*p*(1/L_q-1/L_d)*imag(u_s*psi_s) + 3/2*p/L_d*imag(u_s*psi_r) + k_Te_0;  % 非零电压矢量时转矩变化率

% k = abs((k_Te_1-k_Te_0)/(k_psi_1-k_psi_0))*0.5

g_min = Inf;
best_ratio = 1;

d_Te = 0;
d_psi = 0;

for i=1:n+1
    ratio = (i-1)*1/n;

    Te1_ = Te + Ts*ratio*k_Te_1 + Ts*(1-ratio)*k_Te_0;
    psi1_ = psi + Ts*ratio*k_psi_1 + Ts*(1-ratio)*k_psi_0;

    idid=1/L_d*(V_dq(1)*ratio-R_s*i_s_d+omega*L_q*i_s_q)*Ts;
    iqid=1/L_q*(V_dq(2)*ratio-R_s*i_s_q-omega*(psi_f+L_d*i_s_d))*Ts;
    idnext=i_s_d+idid;
    iqnext=i_s_q+iqid;
    Tenext=3/2*p*iqnext*psi_f;
    Phidnext=L_d*idnext+psi_f;
    Phiqnext=L_q*iqnext;
    Phisnext=(Phidnext*Phidnext+Phiqnext*Phiqnext)^(1/2);

    [i Te1_ Tenext psi1_ Phisnext];

    d_Te = abs(Te_ref - Te1_);
    d_psi = k*abs(psi_ref - abs(psi1_));

    if d_psi>0.02
        continue
    end

    g = d_Te + d_psi;

    if(g < g_min)
        g_min = g;
        best_ratio = ratio;
    end
end

== matlab function DCC_DTC_v5/MATLAB Function ==
  data: Te input; psi_ref output
function psi_ref = fcn(Te)

p = 4;
R_s = 1.2;
L_d = 0.0085;
L_q = 0.0085;
V = 311;
psi_f = 0.175;

psi_ref = sqrt(psi_f^2 + ((2*L_q*Te)/(3*p*psi_f))^2);

== matlab function DCC_DTC_v5/Triggered Subsystem/MATLAB Function ==
  data: Ts input; psi_s_ref input; sa output; Te_ref input; Te input; i_q input; i_d input; omega input; theta input; sb output; sc output
function [sa, sb, sc]  = fcn(Ts, psi_s_ref, Te_ref, Te, i_q, i_d, omega, theta)

R_s       = 1.2;
L_d      = 0.0085;
L_q      = 0.0085;
psi_f    = 0.175;
p       = 4;
V     = 311;
g_min    = Inf;
m       = 50;
i_min    = 1;

sw = [0 0 0; 0 0 1; 0 1 0; 0 1 1; 1 0 0; 1 0 1; 1 1 0; 1 1 1];
trans = 2/3*[cos(theta) cos(theta-2/3*pi) cos(theta+2/3*pi);
             -sin(theta) -sin(theta-2/3*pi) -sin(theta+2/3*pi)];

persistent flag u_d u_q
if isempty(flag)
    flag = 1;
    u_d = 0;
    u_q = 0;
end

%%%%%%%%%%%%%%%%%%%%%%%%%%%%%%%%%%%%%%
% i_s_d = i_d;
% i_s_q = i_q;
% psi_s_d = L_d*i_s_d + psi_f;
% psi_s_q = L_q*i_s_q;
% 
% i_s = i_s_d + 1i*i_s_q;
% psi_s = psi_s_d + 1i*psi_s_q;
% psi_r = psi_f + 1i*0;
% 
% % 计算零电压矢量下变化率
% psi = sqrt(psi_s_d^2 +psi_s_q^2);
% k_psi_0 = -R_s/psi*real(psi_s'*i_s); % 零电压矢量时磁链变化率
% 
% k_Te_0 = -3/2*p*(1/L_q-1/L_d)*omega*real(psi_s^2) + ...
%     3/4*p*R_s*(1/L_d^2-1/L_q^2)*imag(psi_s^2) - ...
%     3/2*p/L_d*(R_s/L_d*imag(psi_s*psi_r) + omega*real(psi_s*psi_r)); % 零电压矢量时转矩变化率
% 
% % 选择电压矢量
% Te1 = Te + k_Te_0*Ts;
% psi1 = psi + k_psi_0*Ts;
%%%%%%%%%%%%%%%%%%%%%%%%%%%%%%%%%%%%%%%%%%%%%%

% i_d1 = i_d+Ts/L_d*(u_d+i_q*omega*L_q-i_d*R_s);
% i_q1 = i_q+Ts/L_q*(u_q-i_d*omega*L_d-i_q*R_s-psi_f*omega);
i_d1 = i_d;
i_q1 = i_q;

for i=1:8
    sa = sw(i,1); sb = sw(i, 2); sc = sw(i, 3);
    Va = V*(2*sa-sb-sc)/3;
    Vb = V*(2*sb-sc-sa)/3;
    Vc = V*(2*sc-sa-sb)/3;
    Vabc = [Va; Vb; Vc];
    V_dq = trans*Vabc;
    V_d = V_dq(1, 1);
    V_q = V_dq(2, 1);
    i_d2 = i_d1+Ts/L_d*(V_d+i_q1*omega*L_q-i_d1*R_s);
    i_q2 = i_q1+Ts/L_q*(V_q-i_d1*omega*L_d-i_q1*R_s-psi_f*omega);
    Te2 = 3/2*p*i_q2*psi_f;
    psi_d2 = L_d*i_d2+psi_f;
    psi_q2 = L_q*i_q2;
    psi_s2 = sqrt(psi_d2^2+psi_q2^2);
    % if i==1
    %     [Te Te1 Te2 psi psi1 psi_s2]
    % elseif i<8
    %     sa = sw(i,1); sb = sw(i, 2); sc = sw(i, 3);
    %     Va = V*(2*sa-sb-sc)/3;
    %     Vb = V*(2*sb-sc-sa)/3;
    %     Vc = V*(2*sc-sa-sb)/3;
    %     Vabc = [Va; Vb; Vc];
    %     the = theta;
    %     trans = 2/3*[cos(the) cos(the-2/3*pi) cos(the+2/3*pi);
    %                  -sin(the) -sin(the-2/3*pi) -sin(the+2/3*pi)];
    %     % trans = 2/3*[sin(the) sin(the-2/3*pi) sin(the+2/3*pi);
    %     %              cos(the) cos(the-2/3*pi) cos(the+2/3*pi)]
    %     V_dq = trans*Vabc;
    %     u_s = V_dq(1) + 1i*V_dq(2);
    %     k_psi_1 = 1/psi*real(psi_s'*u_s) + k_psi_0; % 非零电压矢量时磁链变化率
    %     k_Te_1 = 3/2*p*(1/L_q-1/L_d)*imag(u_s*psi_s) + 3/2*p/L_d*imag(u_s*psi_r) + k_Te_0;  % 非零电压矢量时转矩变化率
    % 
    %     Te1 = Te + Ts*k_Te_1;
    %     psi_s1 = psi + Ts*k_psi_1;
    %     [Te Te1 Te2 psi psi_s1 psi_s2]
    % end
    % if Te2>Te
    %     n = n+1;
    % end
    % if psi_s2 > psi
    %     m = m+1;
    % end
    d_Te = abs(Te_ref - Te2);
    d_psi_s = abs(psi_s_ref-psi_s2);
    g = abs(Te_ref - Te2)+m*abs(psi_s_ref-psi_s2);
    [i g d_Te m*d_psi_s];
    if (g<g_min)
        i_min = i;
        g_min = g;
    end
end

sa = sw(i_min,1); sb = sw(i_min, 2); sc = sw(i_min, 3);
Va = V*(2*sa-sb-sc)/3;
Vb = V*(2*sb-sc-sa)/3;
Vc = V*(2*sc-sa-sb)/3;
Vabc = [Va; Vb; Vc];
V_dq = trans*Vabc;
u_d = V_dq(1, 1);
u_q = V_dq(2, 1);

== matlab function DCC_DTC_v5/Triggered Subsystem1/MATLAB Function ==
  data: Ts input; K input; Tcm1 output; best_ratio input; Tcm2 output; Tcm3 output
function [Tcm1,Tcm2,Tcm3] = fcn(Ts,K,best_ratio)

T1=best_ratio*Ts/2;
T2=T1;
Ta=(Ts-T1-T2)/4;
Tb=Ta+T1/2;
Tc=Tb+T2/2;
Tcm1=1;
Tcm2=1;
Tcm3=1;

if(K==1)
    Tcm1=Tc;Tcm2=Tc;Tcm3=Tc;
end
if(K==2) 
    Tcm1=Ta;Tcm2=Tc;Tcm3=Tc;
end
if(K==3) 
    Tcm1=Ta;Tcm2=Ta;Tcm3=Tc;
end
if(K==4) 
    Tcm1=Tc;Tcm2=Ta;Tcm3=Tc;
end
if(K==5) 
    Tcm1=Tc;Tcm2=Ta;Tcm3=Ta;
end
if(K==6) 
    Tcm1=Tc;Tcm2=Tc;Tcm3=Ta;
end
if(K==7) 
    Tcm1=Ta;Tcm2=Tc;Tcm3=Ta;
end
if(K==8)
    Tcm1=Ta;Tcm2=Ta;Tcm3=Ta;
end
